simulink model "sampleModel44"  (R2021b)
settings: Solver=VariableStepAuto  StartTime=0.0  StopTime=10.0  RelTol=1e-3
undefined symbols (not defined in the file or in its folder): DiscIntNeverNeededParam
libraries: simulink x5
settings Model: Creator=user  LastModifiedBy=user

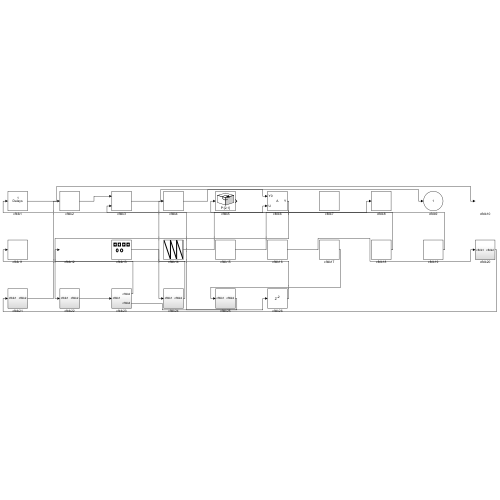
[thumbnail: Simulink's stored preview of the top-level diagram]
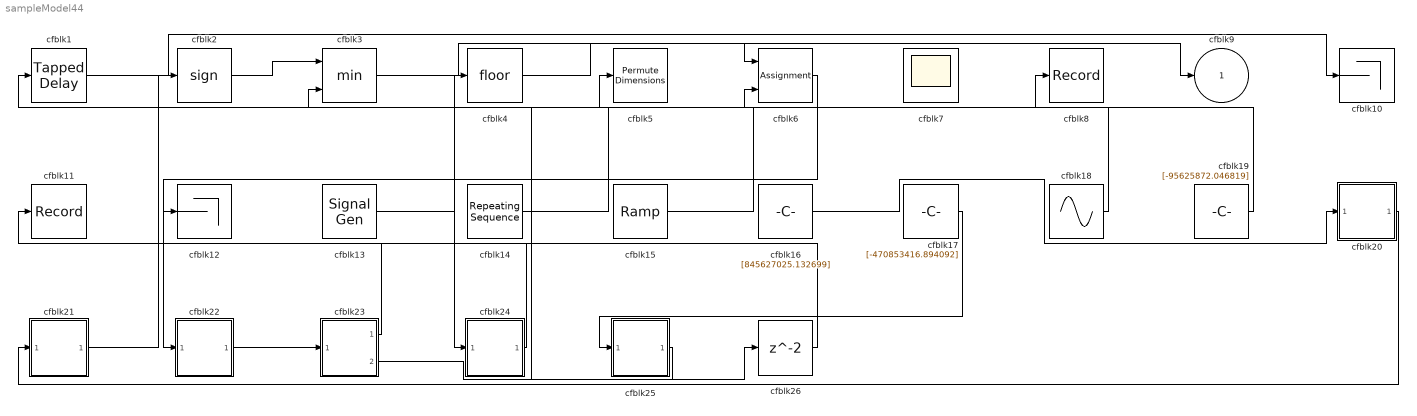
== system sampleModel44 ==
  cfblk1 : simulink/Discrete/Tapped Delay  vinit=0.0  samptime=-1  NumDelays=1  DelayOrder=Oldest  includeCurrent=off
  cfblk10 : Terminator
  cfblk11 : Record  FileSettingsInternal="{\"entries\":[{\"content\":{\"excelSettings\":{\"content\":{},\"type\":\"Streamout.ExcelSettings\"}},\"type\":\"Streamout.FileSettingStorage\",\"uuid\":\"cf80f3d9-e8bc-417e-a10c-4a1480f552fe\"}],\"packageUris\":[\"http://schema.mathworks.com/mf0/streamout_blocks/R2020a\"],\"version\":\"1.0\"}"  SignalsInternal="{\"entries\":[{\"content\":{\"signals\":[{\"content\":{\"blockPath\":[\"sampleModel44/cfblk11\"],\"channel\":[],\"dimensions\":[1],\"domain\":\"sampleModel44/cfblk11\",\"lineColor\":\"#d95319\",\"plots\":[1],\"port\":1,\"sid\":[\"\"],\"signalID\":1707,\"signalName\":\"cfblk24\"},\"type\":\"RecordBlkView.Signal\",\"uuid\":\"c6b62085-c9ed-438e-94d2-a158c6fcdbee\"}]},\"type\":\"RecordBlkView.InputSignals\",\"uuid\":\"0df14473-ce50-43a1-828e-ee86499990f6\"}],\"packageUris\":[\"http://schema.mathworks.com/mf0/streamout_blocks/R2020a\"],\"version\":\"1.0\"}"  VisualizationBindings="{\"sparklinesplugin\":{\"info\":[{\"bindingParametersList\":[],\"subplotID\":1}]}}"
  cfblk12 : Terminator
  cfblk13 : SignalGenerator  WaveForm=square  Amplitude=[756550227.483979]  Units=rad/sec
  cfblk14 : simulink/Sources/Repeating Sequence  rep_seq_t=[0 2]  rep_seq_y=[297071483.694539, 220807238.781131]
  cfblk15 : simulink/Sources/Ramp  slope=[-8220.747417]  start=[18.973469]  InitialOutput=[879904.849925]
  cfblk16 : Constant  Value=[845627025.132699]  SampleTime=1
  cfblk17 : Constant  Value=[-470853416.894092]  SampleTime=1
  cfblk18 : Sin  Amplitude=[-196184416.780537]  Bias=[772911833.250921]  SampleTime=0
  cfblk19 : Constant  Value=[-95625872.046819]  SampleTime=1
  cfblk2 : Signum
  cfblk20 : Subsystem
  cfblk21 : Subsystem
  cfblk22 : Subsystem
  cfblk23 : Subsystem
  cfblk24 : Subsystem
  cfblk25 : Subsystem
  cfblk26 : Delay  SampleTime=1
  cfblk3 : MinMax  Inputs=2
  cfblk4 : Rounding
  cfblk5 : PermuteDimensions
  cfblk6 : Assignment  DiagnosticForDimensions=Warning  IndexOptions=Index vector (dialog)  Indices=1  OutputSizes=1
  cfblk7 : Scope
      settings: Floating=on
  cfblk8 : Record  FileSettingsInternal="{\"entries\":[{\"content\":{\"excelSettings\":{\"content\":{},\"type\":\"Streamout.ExcelSettings\"}},\"type\":\"Streamout.FileSettingStorage\",\"uuid\":\"7597e864-14c6-4c54-930e-17ad618ab8ff\"}],\"packageUris\":[\"http://schema.mathworks.com/mf0/streamout_blocks/R2020a\"],\"version\":\"1.0\"}"  SignalsInternal="{\"entries\":[{\"content\":{\"signals\":[{\"content\":{\"blockPath\":[\"sampleModel44/cfblk8\"],\"channel\":[],\"dimensions\":[1],\"domain\":\"sampleModel44/cfblk8\",\"lineColor\":\"#edb120\",\"plots\":[1],\"port\":1,\"sid\":[\"\"],\"signalID\":1711,\"signalName\":\"cfblk15\"},\"type\":\"RecordBlkView.Signal\",\"uuid\":\"047ba670-b8d1-43b8-b83c-bd241e47a976\"}]},\"type\":\"RecordBlkView.InputSignals\",\"uuid\":\"89e880d1-3009-4126-b160-809cb8ef8eb4\"}],\"packageUris\":[\"http://schema.mathworks.com/mf0/streamout_blocks/R2020a\"],\"version\":\"1.0\"}"  VisualizationBindings="{\"sparklinesplugin\":{\"info\":[{\"bindingParametersList\":[],\"subplotID\":1}]}}"
  cfblk9 : Outport
  wires:
  cfblk17/1 -> cfblk25/1(cfblk1)
  cfblk18/1 -> cfblk5/1
  cfblk24/1(cfblk2) -> cfblk11/1
  cfblk25/1(cfblk2) -> cfblk1/1
  cfblk22/1(cfblk2) -> cfblk23/1(cfblk1)
  cfblk16/1 -> cfblk20/1(cfblk1)
  cfblk2/1 -> cfblk3/1
  cfblk20/1(cfblk2) -> cfblk21/1(cfblk1)
  cfblk19/1 -> cfblk3/2
  cfblk4/1 -> cfblk6/1
  cfblk6/1 -> cfblk22/1(cfblk1)
  cfblk1/1 -> cfblk10/1
  cfblk23/1(cfblk2) -> cfblk12/1
  cfblk14/1 -> cfblk6/2
  cfblk3/1 -> cfblk9/1
  cfblk13/1 -> cfblk24/1(cfblk1)
  cfblk15/1 -> cfblk8/1
  cfblk21/1(cfblk2) -> cfblk2/1
  cfblk23/2(cfblk4) -> cfblk26/1
  cfblk26/1 -> cfblk4/1

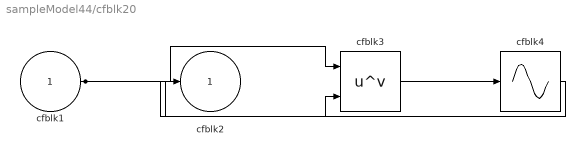
== system sampleModel44/cfblk20 ==
  cfblk1 : Inport
  cfblk3 : Math  Operator=pow  SaturateOnIntegerOverflow=on
  cfblk4 : Sin  TimeSource=Use external signal  SampleTime=0
  cfblk2 : Outport
  wires:
  cfblk1/1 -> cfblk3/1, cfblk3/2
  cfblk3/1 -> cfblk4/1
  cfblk4/1 -> cfblk2/1

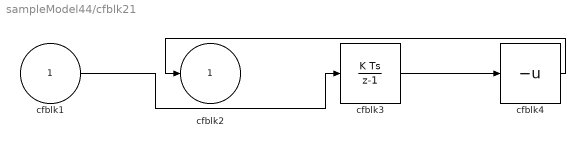
== system sampleModel44/cfblk21 ==
  cfblk1 : Inport
  cfblk3 : DiscreteIntegrator  ICPrevOutput=DiscIntNeverNeededParam  ICPrevScaledInput=DiscIntNeverNeededParam
  cfblk4 : UnaryMinus
  cfblk2 : Outport
  wires:
  cfblk4/1 -> cfblk2/1
  cfblk3/1 -> cfblk4/1
  cfblk1/1 -> cfblk3/1

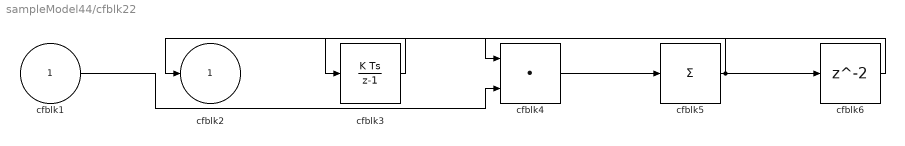
== system sampleModel44/cfblk22 ==
  cfblk1 : Inport
  cfblk3 : DiscreteIntegrator  ICPrevOutput=DiscIntNeverNeededParam  ICPrevScaledInput=DiscIntNeverNeededParam
  cfblk4 : DotProduct  InputSameDT=on  OutDataTypeStr=Inherit: Inherit via internal rule
  cfblk5 : Sum  Inputs=+
  cfblk6 : Delay  SampleTime=1
  cfblk2 : Outport
  wires:
  cfblk3/1 -> cfblk2/1
  cfblk5/1 -> cfblk3/1, cfblk6/1
  cfblk4/1 -> cfblk5/1
  cfblk1/1 -> cfblk4/2
  cfblk6/1 -> cfblk4/1

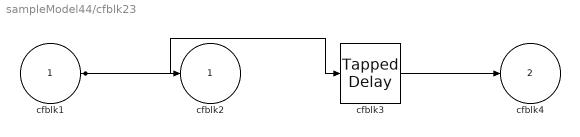
== system sampleModel44/cfblk23 ==
  cfblk1 : Inport
  cfblk3 : simulink/Discrete/Tapped Delay  vinit=0.0  samptime=-1  NumDelays=1  DelayOrder=Oldest  includeCurrent=off
  cfblk2 : Outport
  cfblk4 : Outport  Port=2
  wires:
  cfblk1/1 -> cfblk3/1, cfblk2/1
  cfblk3/1 -> cfblk4/1

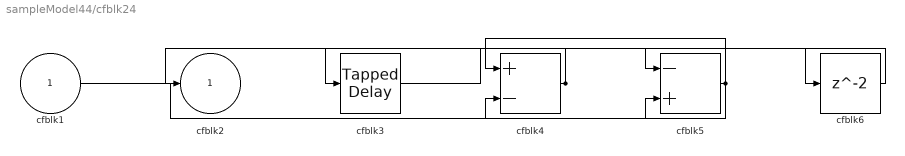
== system sampleModel44/cfblk24 ==
  cfblk1 : Inport
  cfblk3 : simulink/Discrete/Tapped Delay  vinit=0.0  samptime=-1  NumDelays=1  DelayOrder=Oldest  includeCurrent=off
  cfblk4 : Sum  Inputs=+-
  cfblk5 : Sum  Inputs=-+
  cfblk6 : Delay  SampleTime=1
  cfblk2 : Outport
  wires:
  cfblk1/1 -> cfblk5/2
  cfblk5/1 -> cfblk4/1, cfblk4/2
  cfblk4/1 -> cfblk2/1, cfblk3/1
  cfblk3/1 -> cfblk6/1
  cfblk6/1 -> cfblk5/1

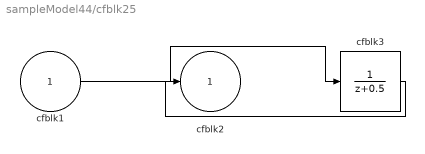
== system sampleModel44/cfblk25 ==
  cfblk1 : Inport
  cfblk3 : DiscreteTransferFcn  SampleTime=1
  cfblk2 : Outport
  wires:
  cfblk1/1 -> cfblk3/1
  cfblk3/1 -> cfblk2/1
